simulink model "Fuzzy_intersection"  (R2025b)
settings: Solver=VariableStepAuto  StartTime=0.0  StopTime=100.0  RelTol=1e-3
model workspace (MAT data in the model file):
  RoadCapacity1 = 10
  RoadCapacity2 = 10
  RoadCapacity3 = 10
  RoadCapacity4 = 10
  TrafficControl : mamfis (value not decoded)
undefined symbols (not defined in the file or in its folder): m, n
libraries: fuzblock x2
settings Model: Creator=gyorgy  LastModifiedBy=gyorgy

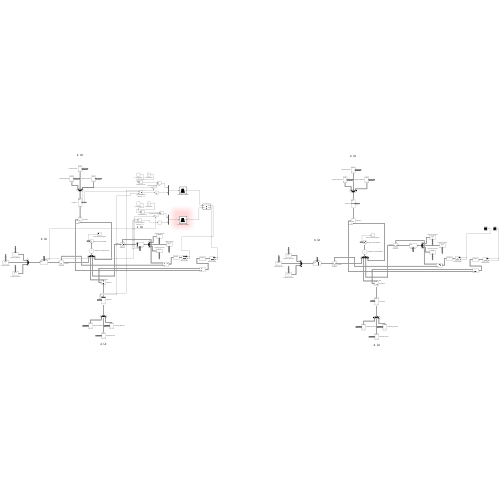
[thumbnail: Simulink's stored preview of the top-level diagram]
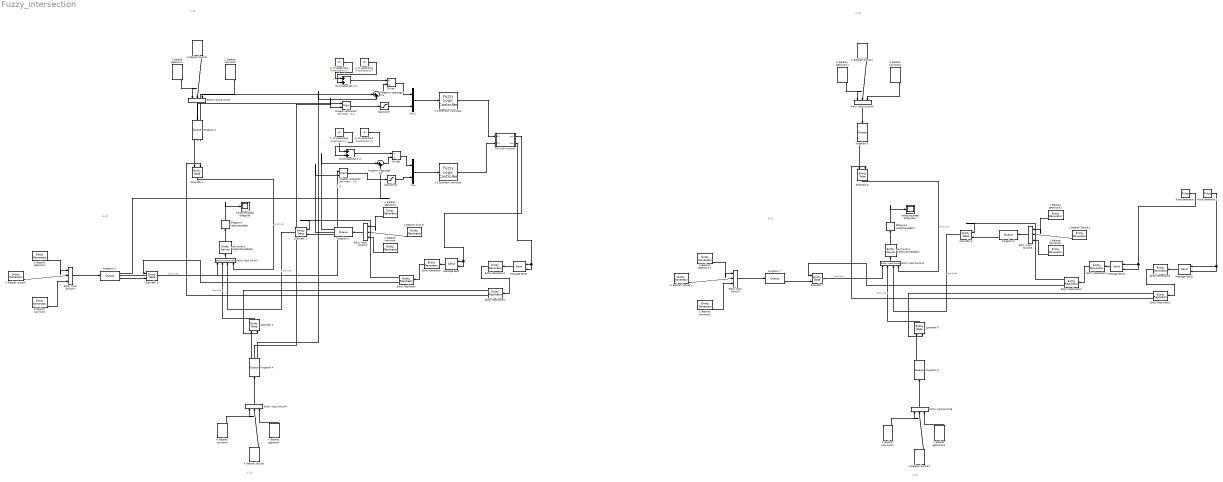
== system Fuzzy_intersection ==
  note: 1. Út
  note: 2. Út
  note: 3. Út
  note: 4. Út
  note: 3. Út
  note: 2. Út
  note: 4. Út
  1-3 Szemafor irányítása : fuzblock/Fuzzy Logic  Controller  FIS=TrafficControl  OutputSampleNumber=101  DataType=double  UseLookupTable=off  NumBreakpoints=10  FuzzifiedInputs=off  RuleFiringStrengths=off  RuleOutputs=off  AggregatedOutputs=off  SimulateUsing=Interpreted execution  OutOfRangeInputValueMessage=warning  NoRuleFiredMessage=warning  EmptyOutputFuzzySetMessage=warning
  1. Bejárat: buszok : EntityGenerator  OutputPortMessageModes=n,n,n,m  TimeSource=MATLAB action  IntergenerationTimeAction=|  GenerateEntityAtSimulationStart=off  GenerateAction=|  AttributeName=Utasok  NumberEntitiesDeparted=on  PendingEntityInBlock=on  AverageIntergenerationTime=on  EntityType=Structured  EntityTypeName=Jarmu
      | persistent rngInit;
      | if isempty(rngInit)
      |     seed = 11111;
      |     rng(seed);
      |     rngInit = true;
      | end
      | a = 1;
      | b = 20;
      | dt = a + (b-a).*rand(1,1);
      | persistent rngInit;
      | if isempty(rngInit)
      |     seed = 11111;
      |     rng(seed);
      |     rngInit = true;
      | end
      | 
      | % Pattern: Gaussian (normal) distribution
      | % m: Mean, d: Standard deviation
      | minpassengers = 1;
      | maxpassengers = 60;
      | m = 0; d = 0.2;
      | entity.Utasok = minpassengers + round((maxpassengers-minpassengers) * abs(m + d * randn));
      settings: OutputPortMap=o0,o1,o2,o3
  1. Bejárat: buszok1 : EntityGenerator  OutputPortMessageModes=n,n,n,m  TimeSource=MATLAB action  IntergenerationTimeAction=|  GenerateEntityAtSimulationStart=off  GenerateAction=|  AttributeName=Utasok  NumberEntitiesDeparted=on  PendingEntityInBlock=on  AverageIntergenerationTime=on  EntityType=Structured  EntityTypeName=Jarmu
      | persistent rngInit;
      | if isempty(rngInit)
      |     seed = 11111;
      |     rng(seed);
      |     rngInit = true;
      | end
      | a = 1;
      | b = 20;
      | dt = a + (b-a).*rand(1,1);
      | persistent rngInit;
      | if isempty(rngInit)
      |     seed = 11111;
      |     rng(seed);
      |     rngInit = true;
      | end
      | 
      | % Pattern: Gaussian (normal) distribution
      | % m: Mean, d: Standard deviation
      | minpassengers = 1;
      | maxpassengers = 60;
      | m = 0; d = 0.2;
      | entity.Utasok = minpassengers + round((maxpassengers-minpassengers) * abs(m + d * randn));
      settings: OutputPortMap=o0,o1,o2,o3
  1. Bejárat: gépkocsik : EntityGenerator  OutputPortMessageModes=n,n,n,m  TimeSource=MATLAB action  Period=0.1  IntergenerationTimeAction=|  GenerateEntityAtSimulationStart=off  GenerateAction=|  AttributeName=Utasok  NumberEntitiesDeparted=on  PendingEntityInBlock=on  AverageIntergenerationTime=on  EntityType=Structured  EntityTypeName=Jarmu
      | persistent rngInit;
      | if isempty(rngInit)
      |     seed = 11111;
      |     rng(seed);
      |     rngInit = true;
      | end
      | a = 1;
      | b = 5;
      | dt = a + (b-a).*rand(1,1);
      | persistent rngInit;
      | if isempty(rngInit)
      |     seed = 11111;
      |     rng(seed);
      |     rngInit = true;
      | end
      | 
      | % Pattern: Gaussian (normal) distribution
      | % m: Mean, d: Standard deviation
      | minpassengers = 1;
      | maxpassengers = 5;
      | m = 0; d = 0.2;
      | entity.Utasok = minpassengers + round((maxpassengers-minpassengers) * abs(m + d * randn));
      settings: OutputPortMap=o0,o1,o2,o3
  1. Bejárat: gépkocsik1 : EntityGenerator  OutputPortMessageModes=n,n,n,m  TimeSource=MATLAB action  Period=0.1  IntergenerationTimeAction=|  GenerateEntityAtSimulationStart=off  GenerateAction=|  AttributeName=Utasok  NumberEntitiesDeparted=on  PendingEntityInBlock=on  AverageIntergenerationTime=on  EntityType=Structured  EntityTypeName=Jarmu
      | persistent rngInit;
      | if isempty(rngInit)
      |     seed = 11111;
      |     rng(seed);
      |     rngInit = true;
      | end
      | a = 1;
      | b = 5;
      | dt = a + (b-a).*rand(1,1);
      | persistent rngInit;
      | if isempty(rngInit)
      |     seed = 11111;
      |     rng(seed);
      |     rngInit = true;
      | end
      | 
      | % Pattern: Gaussian (normal) distribution
      | % m: Mean, d: Standard deviation
      | minpassengers = 1;
      | maxpassengers = 5;
      | m = 0; d = 0.2;
      | entity.Utasok = minpassengers + round((maxpassengers-minpassengers) * abs(m + d * randn));
      settings: OutputPortMap=o0,o1,o2,o3
  1. Bejárat: kamionok : EntityGenerator  OutputPortMessageModes=n,n,n,m  TimeSource=MATLAB action  IntergenerationTimeAction=|  GenerateEntityAtSimulationStart=off  GenerateAction=|  AttributeName=Utasok  NumberEntitiesDeparted=on  PendingEntityInBlock=on  AverageIntergenerationTime=on  EntityType=Structured  EntityTypeName=Jarmu  DataInitialValue=1
      | persistent rngInit;
      | if isempty(rngInit)
      |     seed = 11111;
      |     rng(seed);
      |     rngInit = true;
      | end
      | a = 1;
      | b = 10;
      | dt = a + (b-a).*rand(1,1);
      | persistent rngInit;
      | if isempty(rngInit)
      |     seed = 11111;
      |     rng(seed);
      |     rngInit = true;
      | end
      | 
      | % Pattern: Gaussian (normal) distribution
      | % m: Mean, d: Standard deviation
      | minpassengers = 1;
      | maxpassengers = 2;
      | m = 0; d = 0.2;
      | entity.Utasok = minpassengers + round((maxpassengers-minpassengers) * abs(m + d * randn));
      settings: OutputPortMap=o0,o1,o2,o3
  1. Bejárat: kamionok1 : EntityGenerator  OutputPortMessageModes=n,n,n,m  TimeSource=MATLAB action  IntergenerationTimeAction=|  GenerateEntityAtSimulationStart=off  GenerateAction=|  AttributeName=Utasok  NumberEntitiesDeparted=on  PendingEntityInBlock=on  AverageIntergenerationTime=on  EntityType=Structured  EntityTypeName=Jarmu  DataInitialValue=1
      | persistent rngInit;
      | if isempty(rngInit)
      |     seed = 11111;
      |     rng(seed);
      |     rngInit = true;
      | end
      | a = 1;
      | b = 10;
      | dt = a + (b-a).*rand(1,1);
      | persistent rngInit;
      | if isempty(rngInit)
      |     seed = 11111;
      |     rng(seed);
      |     rngInit = true;
      | end
      | 
      | % Pattern: Gaussian (normal) distribution
      | % m: Mean, d: Standard deviation
      | minpassengers = 1;
      | maxpassengers = 2;
      | m = 0; d = 0.2;
      | entity.Utasok = minpassengers + round((maxpassengers-minpassengers) * abs(m + d * randn));
      settings: OutputPortMap=o0,o1,o2,o3
  "1. út kapacitása " : Constant  Value=RoadCapacity1
  2-4 Szemafor irányítása : fuzblock/Fuzzy Logic  Controller  FIS=TrafficControl  OutputSampleNumber=101  DataType=double  UseLookupTable=off  NumBreakpoints=10  FuzzifiedInputs=off  RuleFiringStrengths=off  RuleOutputs=off  AggregatedOutputs=off  SimulateUsing=Interpreted execution  OutOfRangeInputValueMessage=warning  NoRuleFiredMessage=warning  EmptyOutputFuzzySetMessage=warning
  2. Bejárat: buszok : EntityGenerator  OutputPortMessageModes=n,n,n,m  TimeSource=MATLAB action  IntergenerationTimeAction=|  GenerateEntityAtSimulationStart=off  GenerateAction=|  AttributeName=Utasok  NumberEntitiesDeparted=on  PendingEntityInBlock=on  AverageIntergenerationTime=on  EntityType=Structured  EntityTypeName=Jarmu
      | persistent rngInit;
      | if isempty(rngInit)
      |     seed = 22222;
      |     rng(seed);
      |     rngInit = true;
      | end
      | a = 1;
      | b = 20;
      | dt = a + (b-a).*rand(1,1);
      | persistent rngInit;
      | if isempty(rngInit)
      |     seed = 22222;
      |     rng(seed);
      |     rngInit = true;
      | end
      | 
      | % Pattern: Gaussian (normal) distribution
      | % m: Mean, d: Standard deviation
      | minpassengers = 1;
      | maxpassengers = 60;
      | m = 0; d = 0.2;
      | entity.Utasok = minpassengers + round((maxpassengers-minpassengers) * abs(m + d * randn));
      settings: OutputPortMap=o0,o1,o2,o3
  2. Bejárat: buszok1 : EntityGenerator  OutputPortMessageModes=n,n,n,m  TimeSource=MATLAB action  IntergenerationTimeAction=|  GenerateEntityAtSimulationStart=off  GenerateAction=|  AttributeName=Utasok  NumberEntitiesDeparted=on  PendingEntityInBlock=on  AverageIntergenerationTime=on  EntityType=Structured  EntityTypeName=Jarmu
      | persistent rngInit;
      | if isempty(rngInit)
      |     seed = 22222;
      |     rng(seed);
      |     rngInit = true;
      | end
      | a = 1;
      | b = 20;
      | dt = a + (b-a).*rand(1,1);
      | persistent rngInit;
      | if isempty(rngInit)
      |     seed = 22222;
      |     rng(seed);
      |     rngInit = true;
      | end
      | 
      | % Pattern: Gaussian (normal) distribution
      | % m: Mean, d: Standard deviation
      | minpassengers = 1;
      | maxpassengers = 60;
      | m = 0; d = 0.2;
      | entity.Utasok = minpassengers + round((maxpassengers-minpassengers) * abs(m + d * randn));
      settings: OutputPortMap=o0,o1,o2,o3
  2. Bejárat: gépkocsik : EntityGenerator  OutputPortMessageModes=n,n,n,m  TimeSource=MATLAB action  Period=0.1  IntergenerationTimeAction=|  GenerateEntityAtSimulationStart=off  GenerateAction=|  AttributeName=Utasok  NumberEntitiesDeparted=on  PendingEntityInBlock=on  AverageIntergenerationTime=on  EntityType=Structured  EntityTypeName=Jarmu
      | persistent rngInit;
      | if isempty(rngInit)
      |     seed = 22222;
      |     rng(seed);
      |     rngInit = true;
      | end
      | a = 1;
      | b = 5;
      | dt = a + (b-a).*rand(1,1);
      | persistent rngInit;
      | if isempty(rngInit)
      |     seed = 22222;
      |     rng(seed);
      |     rngInit = true;
      | end
      | 
      | % Pattern: Gaussian (normal) distribution
      | % m: Mean, d: Standard deviation
      | minpassengers = 1;
      | maxpassengers = 5;
      | m = 0; d = 0.2;
      | entity.Utasok = minpassengers + round((maxpassengers-minpassengers) * abs(m + d * randn));
      settings: OutputPortMap=o0,o1,o2,o3
  2. Bejárat: gépkocsik1 : EntityGenerator  OutputPortMessageModes=n,n,n,m  TimeSource=MATLAB action  Period=0.1  IntergenerationTimeAction=|  GenerateEntityAtSimulationStart=off  GenerateAction=|  AttributeName=Utasok  NumberEntitiesDeparted=on  PendingEntityInBlock=on  AverageIntergenerationTime=on  EntityType=Structured  EntityTypeName=Jarmu
      | persistent rngInit;
      | if isempty(rngInit)
      |     seed = 22222;
      |     rng(seed);
      |     rngInit = true;
      | end
      | a = 1;
      | b = 5;
      | dt = a + (b-a).*rand(1,1);
      | persistent rngInit;
      | if isempty(rngInit)
      |     seed = 22222;
      |     rng(seed);
      |     rngInit = true;
      | end
      | 
      | % Pattern: Gaussian (normal) distribution
      | % m: Mean, d: Standard deviation
      | minpassengers = 1;
      | maxpassengers = 5;
      | m = 0; d = 0.2;
      | entity.Utasok = minpassengers + round((maxpassengers-minpassengers) * abs(m + d * randn));
      settings: OutputPortMap=o0,o1,o2,o3
  2. Bejárat: kamionok : EntityGenerator  OutputPortMessageModes=n,n,n,m  TimeSource=MATLAB action  IntergenerationTimeAction=|  GenerateEntityAtSimulationStart=off  GenerateAction=|  AttributeName=Utasok  NumberEntitiesDeparted=on  PendingEntityInBlock=on  AverageIntergenerationTime=on  EntityType=Structured  EntityTypeName=Jarmu
      | persistent rngInit;
      | if isempty(rngInit)
      |     seed = 22222;
      |     rng(seed);
      |     rngInit = true;
      | end
      | a = 1;
      | b = 10;
      | dt = a + (b-a).*rand(1,1);
      | persistent rngInit;
      | if isempty(rngInit)
      |     seed = 22222;
      |     rng(seed);
      |     rngInit = true;
      | end
      | 
      | % Pattern: Gaussian (normal) distribution
      | % m: Mean, d: Standard deviation
      | minpassengers = 1;
      | maxpassengers = 2;
      | m = 0; d = 0.2;
      | entity.Utasok = minpassengers + round((maxpassengers-minpassengers) * abs(m + d * randn));
      settings: OutputPortMap=o0,o1,o2,o3
  2. Bejárat: kamionok1 : EntityGenerator  OutputPortMessageModes=n,n,n,m  TimeSource=MATLAB action  IntergenerationTimeAction=|  GenerateEntityAtSimulationStart=off  GenerateAction=|  AttributeName=Utasok  NumberEntitiesDeparted=on  PendingEntityInBlock=on  AverageIntergenerationTime=on  EntityType=Structured  EntityTypeName=Jarmu
      | persistent rngInit;
      | if isempty(rngInit)
      |     seed = 22222;
      |     rng(seed);
      |     rngInit = true;
      | end
      | a = 1;
      | b = 10;
      | dt = a + (b-a).*rand(1,1);
      | persistent rngInit;
      | if isempty(rngInit)
      |     seed = 22222;
      |     rng(seed);
      |     rngInit = true;
      | end
      | 
      | % Pattern: Gaussian (normal) distribution
      | % m: Mean, d: Standard deviation
      | minpassengers = 1;
      | maxpassengers = 2;
      | m = 0; d = 0.2;
      | entity.Utasok = minpassengers + round((maxpassengers-minpassengers) * abs(m + d * randn));
      settings: OutputPortMap=o0,o1,o2,o3
  2. út kapacitása : Constant  Value=RoadCapacity2
  3. Bejárat: buszok : EntityGenerator  OutputPortMessageModes=n,n,n,m  TimeSource=MATLAB action  IntergenerationTimeAction=|  GenerateEntityAtSimulationStart=off  GenerateAction=|  AttributeName=Utasok  NumberEntitiesDeparted=on  PendingEntityInBlock=on  AverageIntergenerationTime=on  EntityType=Structured  EntityTypeName=Jarmu
      | persistent rngInit;
      | if isempty(rngInit)
      |     seed = 33333;
      |     rng(seed);
      |     rngInit = true;
      | end
      | a = 1;
      | b = 20;
      | dt = a + (b-a).*rand(1,1);
      | persistent rngInit;
      | if isempty(rngInit)
      |     seed = 33333;
      |     rng(seed);
      |     rngInit = true;
      | end
      | 
      | % Pattern: Gaussian (normal) distribution
      | % m: Mean, d: Standard deviation
      | minpassengers = 1;
      | maxpassengers = 60;
      | m = 0; d = 0.2;
      | entity.Utasok = minpassengers + round((maxpassengers-minpassengers) * abs(m + d * randn));
      settings: OutputPortMap=o0,o1,o2,o3
  3. Bejárat: buszok1 : EntityGenerator  OutputPortMessageModes=n,n,n,m  TimeSource=MATLAB action  IntergenerationTimeAction=|  GenerateEntityAtSimulationStart=off  GenerateAction=|  AttributeName=Utasok  NumberEntitiesDeparted=on  PendingEntityInBlock=on  AverageIntergenerationTime=on  EntityType=Structured  EntityTypeName=Jarmu
      | persistent rngInit;
      | if isempty(rngInit)
      |     seed = 33333;
      |     rng(seed);
      |     rngInit = true;
      | end
      | a = 1;
      | b = 20;
      | dt = a + (b-a).*rand(1,1);
      | persistent rngInit;
      | if isempty(rngInit)
      |     seed = 33333;
      |     rng(seed);
      |     rngInit = true;
      | end
      | 
      | % Pattern: Gaussian (normal) distribution
      | % m: Mean, d: Standard deviation
      | minpassengers = 1;
      | maxpassengers = 60;
      | m = 0; d = 0.2;
      | entity.Utasok = minpassengers + round((maxpassengers-minpassengers) * abs(m + d * randn));
      settings: OutputPortMap=o0,o1,o2,o3
  3. Bejárat: gépkocsik : EntityGenerator  OutputPortMessageModes=n,n,n,m  TimeSource=MATLAB action  Period=0.1  IntergenerationTimeAction=|  GenerateEntityAtSimulationStart=off  GenerateAction=|  AttributeName=Utasok  NumberEntitiesDeparted=on  PendingEntityInBlock=on  AverageIntergenerationTime=on  EntityType=Structured  EntityTypeName=Jarmu
      | persistent rngInit;
      | if isempty(rngInit)
      |     seed = 33333;
      |     rng(seed);
      |     rngInit = true;
      | end
      | a = 1;
      | b = 5;
      | dt = a + (b-a).*rand(1,1);
      | persistent rngInit;
      | if isempty(rngInit)
      |     seed = 33333;
      |     rng(seed);
      |     rngInit = true;
      | end
      | 
      | % Pattern: Gaussian (normal) distribution
      | % m: Mean, d: Standard deviation
      | minpassengers = 1;
      | maxpassengers = 5;
      | m = 0; d = 0.2;
      | entity.Utasok = minpassengers + round((maxpassengers-minpassengers) * abs(m + d * randn));
      settings: OutputPortMap=o0,o1,o2,o3
  3. Bejárat: gépkocsik1 : EntityGenerator  OutputPortMessageModes=n,n,n,m  TimeSource=MATLAB action  Period=0.1  IntergenerationTimeAction=|  GenerateEntityAtSimulationStart=off  GenerateAction=|  AttributeName=Utasok  NumberEntitiesDeparted=on  PendingEntityInBlock=on  AverageIntergenerationTime=on  EntityType=Structured  EntityTypeName=Jarmu
      | persistent rngInit;
      | if isempty(rngInit)
      |     seed = 33333;
      |     rng(seed);
      |     rngInit = true;
      | end
      | a = 1;
      | b = 5;
      | dt = a + (b-a).*rand(1,1);
      | persistent rngInit;
      | if isempty(rngInit)
      |     seed = 33333;
      |     rng(seed);
      |     rngInit = true;
      | end
      | 
      | % Pattern: Gaussian (normal) distribution
      | % m: Mean, d: Standard deviation
      | minpassengers = 1;
      | maxpassengers = 5;
      | m = 0; d = 0.2;
      | entity.Utasok = minpassengers + round((maxpassengers-minpassengers) * abs(m + d * randn));
      settings: OutputPortMap=o0,o1,o2,o3
  3. Bejárat: kamionok : EntityGenerator  OutputPortMessageModes=n,n,n,m  TimeSource=MATLAB action  IntergenerationTimeAction=|  GenerateEntityAtSimulationStart=off  GenerateAction=|  AttributeName=Utasok  NumberEntitiesDeparted=on  PendingEntityInBlock=on  AverageIntergenerationTime=on  EntityType=Structured  EntityTypeName=Jarmu
      | persistent rngInit;
      | if isempty(rngInit)
      |     seed = 33333;
      |     rng(seed);
      |     rngInit = true;
      | end
      | a = 1;
      | b = 10;
      | dt = a + (b-a).*rand(1,1);
      | persistent rngInit;
      | if isempty(rngInit)
      |     seed = 33333;
      |     rng(seed);
      |     rngInit = true;
      | end
      | 
      | % Pattern: Gaussian (normal) distribution
      | % m: Mean, d: Standard deviation
      | minpassengers = 1;
      | maxpassengers = 2;
      | m = 0; d = 0.2;
      | entity.Utasok = minpassengers + round((maxpassengers-minpassengers) * abs(m + d * randn));
      settings: OutputPortMap=o0,o1,o2,o3
  3. Bejárat: kamionok1 : EntityGenerator  OutputPortMessageModes=n,n,n,m  TimeSource=MATLAB action  IntergenerationTimeAction=|  GenerateEntityAtSimulationStart=off  GenerateAction=|  AttributeName=Utasok  NumberEntitiesDeparted=on  PendingEntityInBlock=on  AverageIntergenerationTime=on  EntityType=Structured  EntityTypeName=Jarmu
      | persistent rngInit;
      | if isempty(rngInit)
      |     seed = 33333;
      |     rng(seed);
      |     rngInit = true;
      | end
      | a = 1;
      | b = 10;
      | dt = a + (b-a).*rand(1,1);
      | persistent rngInit;
      | if isempty(rngInit)
      |     seed = 33333;
      |     rng(seed);
      |     rngInit = true;
      | end
      | 
      | % Pattern: Gaussian (normal) distribution
      | % m: Mean, d: Standard deviation
      | minpassengers = 1;
      | maxpassengers = 2;
      | m = 0; d = 0.2;
      | entity.Utasok = minpassengers + round((maxpassengers-minpassengers) * abs(m + d * randn));
      settings: OutputPortMap=o0,o1,o2,o3
  3. út kapacitása : Constant  Value=RoadCapacity3
  4. Bejárat: buszok : EntityGenerator  OutputPortMessageModes=n,n,n,m  TimeSource=MATLAB action  IntergenerationTimeAction=|  GenerateEntityAtSimulationStart=off  GenerateAction=|  AttributeName=Utasok  NumberEntitiesDeparted=on  PendingEntityInBlock=on  AverageIntergenerationTime=on  EntityType=Structured  EntityTypeName=Jarmu
      | persistent rngInit;
      | if isempty(rngInit)
      |     seed = 44444;
      |     rng(seed);
      |     rngInit = true;
      | end
      | a = 1;
      | b = 20;
      | dt = a + (b-a).*rand(1,1);
      | persistent rngInit;
      | if isempty(rngInit)
      |     seed = 44444;
      |     rng(seed);
      |     rngInit = true;
      | end
      | 
      | % Pattern: Gaussian (normal) distribution
      | % m: Mean, d: Standard deviation
      | minpassengers = 1;
      | maxpassengers = 60;
      | m = 0; d = 0.2;
      | entity.Utasok = minpassengers + round((maxpassengers-minpassengers) * abs(m + d * randn));
      settings: OutputPortMap=o0,o1,o2,o3
  4. Bejárat: buszok1 : EntityGenerator  OutputPortMessageModes=n,n,n,m  TimeSource=MATLAB action  IntergenerationTimeAction=|  GenerateEntityAtSimulationStart=off  GenerateAction=|  AttributeName=Utasok  NumberEntitiesDeparted=on  PendingEntityInBlock=on  AverageIntergenerationTime=on  EntityType=Structured  EntityTypeName=Jarmu
      | persistent rngInit;
      | if isempty(rngInit)
      |     seed = 44444;
      |     rng(seed);
      |     rngInit = true;
      | end
      | a = 1;
      | b = 20;
      | dt = a + (b-a).*rand(1,1);
      | persistent rngInit;
      | if isempty(rngInit)
      |     seed = 44444;
      |     rng(seed);
      |     rngInit = true;
      | end
      | 
      | % Pattern: Gaussian (normal) distribution
      | % m: Mean, d: Standard deviation
      | minpassengers = 1;
      | maxpassengers = 60;
      | m = 0; d = 0.2;
      | entity.Utasok = minpassengers + round((maxpassengers-minpassengers) * abs(m + d * randn));
      settings: OutputPortMap=o0,o1,o2,o3
  4. Bejárat: gépkocsik : EntityGenerator  OutputPortMessageModes=n,n,n,m  TimeSource=MATLAB action  Period=0.1  IntergenerationTimeAction=|  GenerateEntityAtSimulationStart=off  GenerateAction=|  AttributeName=Utasok  NumberEntitiesDeparted=on  PendingEntityInBlock=on  AverageIntergenerationTime=on  EntityType=Structured  EntityTypeName=Jarmu
      | persistent rngInit;
      | if isempty(rngInit)
      |     seed = 44444;
      |     rng(seed);
      |     rngInit = true;
      | end
      | a = 1;
      | b = 5;
      | dt = a + (b-a).*rand(1,1);
      | persistent rngInit;
      | if isempty(rngInit)
      |     seed = 44444;
      |     rng(seed);
      |     rngInit = true;
      | end
      | 
      | % Pattern: Gaussian (normal) distribution
      | % m: Mean, d: Standard deviation
      | minpassengers = 1;
      | maxpassengers = 5;
      | m = 0; d = 0.2;
      | entity.Utasok = minpassengers + round((maxpassengers-minpassengers) * abs(m + d * randn));
      settings: OutputPortMap=o0,o1,o2,o3
  4. Bejárat: gépkocsik1 : EntityGenerator  OutputPortMessageModes=n,n,n,m  TimeSource=MATLAB action  Period=0.1  IntergenerationTimeAction=|  GenerateEntityAtSimulationStart=off  GenerateAction=|  AttributeName=Utasok  NumberEntitiesDeparted=on  PendingEntityInBlock=on  AverageIntergenerationTime=on  EntityType=Structured  EntityTypeName=Jarmu
      | persistent rngInit;
      | if isempty(rngInit)
      |     seed = 44444;
      |     rng(seed);
      |     rngInit = true;
      | end
      | a = 1;
      | b = 5;
      | dt = a + (b-a).*rand(1,1);
      | persistent rngInit;
      | if isempty(rngInit)
      |     seed = 44444;
      |     rng(seed);
      |     rngInit = true;
      | end
      | 
      | % Pattern: Gaussian (normal) distribution
      | % m: Mean, d: Standard deviation
      | minpassengers = 1;
      | maxpassengers = 5;
      | m = 0; d = 0.2;
      | entity.Utasok = minpassengers + round((maxpassengers-minpassengers) * abs(m + d * randn));
      settings: OutputPortMap=o0,o1,o2,o3
  4. Bejárat: kamionok : EntityGenerator  OutputPortMessageModes=n,n,n,m  TimeSource=MATLAB action  IntergenerationTimeAction=|  GenerateEntityAtSimulationStart=off  GenerateAction=|  AttributeName=Utasok  NumberEntitiesDeparted=on  PendingEntityInBlock=on  AverageIntergenerationTime=on  EntityType=Structured  EntityTypeName=Jarmu
      | persistent rngInit;
      | if isempty(rngInit)
      |     seed = 44444;
      |     rng(seed);
      |     rngInit = true;
      | end
      | a = 1;
      | b = 10;
      | dt = a + (b-a).*rand(1,1);
      | persistent rngInit;
      | if isempty(rngInit)
      |     seed = 44444;
      |     rng(seed);
      |     rngInit = true;
      | end
      | 
      | % Pattern: Gaussian (normal) distribution
      | % m: Mean, d: Standard deviation
      | minpassengers = 1;
      | maxpassengers = 2;
      | m = 0; d = 0.2;
      | entity.Utasok = minpassengers + round((maxpassengers-minpassengers) * abs(m + d * randn));
      settings: OutputPortMap=o0,o1,o2,o3
  4. Bejárat: kamionok1 : EntityGenerator  OutputPortMessageModes=n,n,n,m  TimeSource=MATLAB action  IntergenerationTimeAction=|  GenerateEntityAtSimulationStart=off  GenerateAction=|  AttributeName=Utasok  NumberEntitiesDeparted=on  PendingEntityInBlock=on  AverageIntergenerationTime=on  EntityType=Structured  EntityTypeName=Jarmu
      | persistent rngInit;
      | if isempty(rngInit)
      |     seed = 44444;
      |     rng(seed);
      |     rngInit = true;
      | end
      | a = 1;
      | b = 10;
      | dt = a + (b-a).*rand(1,1);
      | persistent rngInit;
      | if isempty(rngInit)
      |     seed = 44444;
      |     rng(seed);
      |     rngInit = true;
      | end
      | 
      | % Pattern: Gaussian (normal) distribution
      | % m: Mean, d: Standard deviation
      | minpassengers = 1;
      | maxpassengers = 2;
      | m = 0; d = 0.2;
      | entity.Utasok = minpassengers + round((maxpassengers-minpassengers) * abs(m + d * randn));
      settings: OutputPortMap=o0,o1,o2,o3
  4. út kapacitása : Constant  Value=RoadCapacity4
  Atlagos várakozási idő (max) - 1-3 : MinMax  Function=max  Inputs=2
  Atlagos várakozási idő (max) - 2-4 : MinMax  Function=max  Inputs=2  OutDataTypeStr=double
  Divide : Product  Inputs=/*
  Divide1 : Product  Inputs=/*  InputSameDT=on  OutDataTypeStr=double
  Elhagyja a kereszteződést : EntityTerminator  InputPortMessageModes=m  NumberEntitiesArrived=on
      settings: OutputPortMap=o0
  Elhagyja a kereszteződést1 : EntityTerminator  InputPortMessageModes=m  NumberEntitiesArrived=on
      settings: OutputPortMap=o0
  Entity Input Switch : EntityInputSwitch  InputPortMessageModes=m,m,m,m  OutputPortMessageModes=m  NumberInputPorts=4
      settings: InputPortMap=u1,u2,u3,u4
  Entity Input Switch1 : EntityInputSwitch  InputPortMessageModes=m,m,m,m  OutputPortMessageModes=m  NumberInputPorts=4
      settings: InputPortMap=u1,u2,u3,u4
  Entity Input Switch{2..9} (8 alike) : EntityInputSwitch  InputPortMessageModes=m,m,m  OutputPortMessageModes=m  NumberInputPorts=3
      settings: InputPortMap=u1,u2,u3
  Entity Generator{,1..3} (4 alike) : EntityGenerator  InputPortMessageModes=m  OutputPortMessageModes=m  GenerationMethod=Event-based  TimeSource=Signal port  AttributeName=entity  EntityTypeName=Entity  DataInitialValue=1
      settings: InputPortMap=u0
  Entity Replicator : EntityReplicator  InputPortMessageModes=m  OutputPortMessageModes=m,m  ReplicasDepartFrom=Single output port  NumberReplicas=2  HoldOriginalEntityUntilAllReplicasDepart=on
  Entity Replicator1 : EntityReplicator  InputPortMessageModes=m  OutputPortMessageModes=m,m  ReplicasDepartFrom=Single output port  NumberReplicas=2
  Entity Replicator2 : EntityReplicator  InputPortMessageModes=m  OutputPortMessageModes=m,m  ReplicasDepartFrom=Single output port  NumberReplicas=2  HoldOriginalEntityUntilAllReplicasDepart=on
  Entity Replicator3 : EntityReplicator  InputPortMessageModes=m  OutputPortMessageModes=m,m  ReplicasDepartFrom=Single output port  NumberReplicas=2
  Forgalom 1 : Queue  InputPortMessageModes=m  OutputPortMessageModes=n,n,m  Capacity=RoadCapacity1  NumberEntitiesInBlock=on  AverageWait=on
      settings: OutputPortMap=o1,o2,o5
  Forgalom 2 : Queue  InputPortMessageModes=m  OutputPortMessageModes=n,n,m  Capacity=RoadCapacity2  NumberEntitiesInBlock=on  AverageWait=on
      settings: OutputPortMap=o1,o2,o5
  Forgalom 3 : Queue  InputPortMessageModes=m  OutputPortMessageModes=n,n,m  Capacity=RoadCapacity3  NumberEntitiesInBlock=on  AverageWait=on
      settings: OutputPortMap=o1,o2,o5
  Forgalom 4 : Queue  InputPortMessageModes=m  OutputPortMessageModes=n,n,m  Capacity=RoadCapacity4  NumberEntitiesInBlock=on  AverageWait=on
      settings: OutputPortMap=o1,o2,o5
  Forgalom 5 : Queue  InputPortMessageModes=m  OutputPortMessageModes=n,n,m  Capacity=RoadCapacity1  NumberEntitiesInBlock=on  AverageWait=on
      settings: OutputPortMap=o1,o2,o5
  Forgalom 6 : Queue  InputPortMessageModes=m  OutputPortMessageModes=n,n,m  Capacity=RoadCapacity2  NumberEntitiesInBlock=on  AverageWait=on
      settings: OutputPortMap=o1,o2,o5
  Forgalom 7 : Queue  InputPortMessageModes=m  OutputPortMessageModes=n,n,m  Capacity=RoadCapacity3  NumberEntitiesInBlock=on  AverageWait=on
      settings: OutputPortMap=o1,o2,o5
  Forgalom 8 : Queue  InputPortMessageModes=m  OutputPortMessageModes=n,n,m  Capacity=RoadCapacity4  NumberEntitiesInBlock=on  AverageWait=on
      settings: OutputPortMap=o1,o2,o5
  Forgalom nagysága - 1-3 : Sum  Inputs=|++
  Forgalom nagysága - 2-4 : Sum  Inputs=|++
  Járművek a keresztezodésben : EntityServer  InputPortMessageModes=m  OutputPortMessageModes=m  Capacity=2  ServiceTimeSource=MATLAB action  ServiceTimeAction=|
      | persistent rngInit;
      | if isempty(rngInit)
      |     seed = 55555;
      |     rng(seed);
      |     rngInit = true;
      | end
      | 
      | % Pattern: Gaussian (normal) distribution
      | % m: Mean, d: Standard deviation
      | m = 0; d = 1;
      | dt = abs(m + d * randn);
  Járművek a keresztezodésben1 : EntityServer  InputPortMessageModes=m  OutputPortMessageModes=m  Capacity=2  ServiceTimeSource=MATLAB action  ServiceTimeAction=|
      | persistent rngInit;
      | if isempty(rngInit)
      |     seed = 55555;
      |     rng(seed);
      |     rngInit = true;
      | end
      | 
      | % Pattern: Gaussian (normal) distribution
      | % m: Mean, d: Standard deviation
      | m = 0; d = 1;
      | dt = abs(m + d * randn);
  Kereszteződést elhagyták : Scope
      settings: ActiveDisplayYMinimum=227.06108147411885  ActiveDisplayYMaximum=238.86097723623857
  Kereszteződést elhagyták1 : Scope
      settings: ActiveDisplayYMinimum=222.88265852629056  ActiveDisplayYMaximum=223.04054883446648
  MATLAB Function : MATLAB Function  TreatAsAtomicUnit=on
  Message Send{,1..3} (4 alike) : Send  OutputPortMessageModes=m  ShowEnablePort=on
      settings: InputPortMap=e0,u1
  Mux : Mux  Inputs=2
  Mux1 : Mux  Inputs=2
  Pulse Generator : DiscretePulseGenerator  PulseType=Time based  Period=20  PulseWidth=50
  Pulse Generator1 : DiscretePulseGenerator  PulseType=Time based  Period=20  PulseWidth=50  PhaseDelay=10
  Saturation : Saturate  UpperLimit=30  LowerLimit=0  OutDataTypeStr=double
  Saturation1 : Saturate  UpperLimit=30  LowerLimit=0  OutDataTypeStr=double
  Szemafor {1..8} (8 alike) : EntityGate  InputPortMessageModes=m,m  OutputPortMessageModes=m
  Összkapacitás 1-3 : Sum
  Összkapacitás 2-4 : Sum
  wires:
  Forgalom 1/3 -> Szemafor 1/2
  Forgalom 2/3 -> Szemafor 2/2
  Forgalom 3/3 -> Szemafor 3/2
  Entity Input Switch3/1 -> Forgalom 3/1
  Forgalom 4/3 -> Szemafor 4/2
  Entity Input Switch4/1 -> Forgalom 4/1
  Járművek a keresztezodésben/1 -> Elhagyja a kereszteződést/1
  Entity Input Switch/1 -> Járművek a keresztezodésben/1
  Szemafor 3/1 -> Entity Input Switch/1  "Járművek"
  Szemafor 4/1 -> Entity Input Switch/2  "Járművek"
  Szemafor 1/1 -> Entity Input Switch/3  "Járművek"
  Szemafor 2/1 -> Entity Input Switch/4  "Járművek"
  Entity Input Switch5/1 -> Forgalom 2/1
  1. Bejárat: gépkocsik/4 -> Entity Input Switch2/1
  1. Bejárat: buszok/4 -> Entity Input Switch2/2
  1. Bejárat: kamionok/4 -> Entity Input Switch2/3
  2. Bejárat: kamionok/4 -> Entity Input Switch5/3
  2. Bejárat: gépkocsik/4 -> Entity Input Switch5/1
  2. Bejárat: buszok/4 -> Entity Input Switch5/2
  3. Bejárat: buszok/4 -> Entity Input Switch3/2
  3. Bejárat: gépkocsik/4 -> Entity Input Switch3/1
  3. Bejárat: kamionok/4 -> Entity Input Switch3/3
  4. Bejárat: buszok/4 -> Entity Input Switch4/2
  4. Bejárat: gépkocsik/4 -> Entity Input Switch4/3
  4. Bejárat: kamionok/4 -> Entity Input Switch4/1
  Mux/1 -> 1-3 Szemafor irányítása/1
  Forgalom 1/2 -> Atlagos várakozási idő (max) - 1-3/2
  Forgalom 3/2 -> Atlagos várakozási idő (max) - 1-3/1
  Mux1/1 -> 2-4 Szemafor irányítása/1
  Forgalom 1/1 -> Forgalom nagysága - 1-3/1
  Forgalom 3/1 -> Forgalom nagysága - 1-3/2
  Forgalom 4/1 -> Forgalom nagysága - 2-4/2
  Forgalom 2/1 -> Forgalom nagysága - 2-4/1
  Entity Replicator/1 -> Szemafor 1/1
  Entity Replicator/2 -> Szemafor 3/1
  Entity Replicator1/1 -> Szemafor 4/1
  Entity Replicator1/2 -> Szemafor 2/1
  Entity Input Switch2/1 -> Forgalom 1/1
  Saturation/1 -> Mux1/2
  Saturation1/1 -> Mux/2
  Atlagos várakozási idő (max) - 1-3/1 -> Saturation1/1
  2. út kapacitása/1 -> Összkapacitás 2-4/1
  4. út kapacitása/1 -> Összkapacitás 2-4/2
  "1. út kapacitása "/1 -> Összkapacitás 1-3/1
  3. út kapacitása/1 -> Összkapacitás 1-3/2
  Forgalom nagysága - 2-4/1 -> Divide/2
  Összkapacitás 1-3/1 -> Divide1/1
  Divide1/1 -> Mux/1
  Összkapacitás 2-4/1 -> Divide/1
  Divide/1 -> Mux1/1
  Atlagos várakozási idő (max) - 2-4/1 -> Saturation/1
  Forgalom nagysága - 1-3/1 -> Divide1/2
  Forgalom 4/2 -> Atlagos várakozási idő (max) - 2-4/2
  Forgalom 2/2 -> Atlagos várakozási idő (max) - 2-4/1
  Entity Generator/1 -> Entity Replicator/1
  Entity Generator1/1 -> Entity Replicator1/1
  Message Send/1 -> Entity Generator/1
  MATLAB Function/1(sig1) -> Message Send/1, Message Send/2
  Message Send1/1 -> Entity Generator1/1
  MATLAB Function/2(sig2) -> Message Send1/1, Message Send1/2
  Elhagyja a kereszteződést/1 -> Kereszteződést elhagyták/1
  4. Bejárat: buszok1/4 -> Entity Input Switch8/2
  Járművek a keresztezodésben1/1 -> Elhagyja a kereszteződést1/1
  2. Bejárat: kamionok1/4 -> Entity Input Switch9/3
  2. Bejárat: gépkocsik1/4 -> Entity Input Switch9/1
  3. Bejárat: kamionok1/4 -> Entity Input Switch7/3
  Forgalom 5/3 -> Szemafor 5/2
  Entity Replicator3/1 -> Szemafor 8/1
  Entity Input Switch8/1 -> Forgalom 8/1
  Entity Replicator2/2 -> Szemafor 7/1
  1. Bejárat: kamionok1/4 -> Entity Input Switch6/3
  1. Bejárat: buszok1/4 -> Entity Input Switch6/2
  2. Bejárat: buszok1/4 -> Entity Input Switch9/2
  Entity Input Switch9/1 -> Forgalom 6/1
  Entity Input Switch1/1 -> Járművek a keresztezodésben1/1
  1. Bejárat: gépkocsik1/4 -> Entity Input Switch6/1
  4. Bejárat: gépkocsik1/4 -> Entity Input Switch8/3
  Szemafor 7/1 -> Entity Input Switch1/1  "Járművek"
  Entity Replicator2/1 -> Szemafor 5/1
  Message Send3/1 -> Entity Generator3/1
  3. Bejárat: gépkocsik1/4 -> Entity Input Switch7/1
  Forgalom 6/3 -> Szemafor 6/2
  Entity Input Switch6/1 -> Forgalom 5/1
  Szemafor 5/1 -> Entity Input Switch1/3  "Járművek"
  4. Bejárat: kamionok1/4 -> Entity Input Switch8/1
  Forgalom 8/3 -> Szemafor 8/2
  Message Send2/1 -> Entity Generator2/1
  Elhagyja a kereszteződést1/1 -> Kereszteződést elhagyták1/1
  Entity Input Switch7/1 -> Forgalom 7/1
  3. Bejárat: buszok1/4 -> Entity Input Switch7/2
  Entity Replicator3/2 -> Szemafor 6/1
  Forgalom 7/3 -> Szemafor 7/2
  Szemafor 8/1 -> Entity Input Switch1/2  "Járművek"
  Szemafor 6/1 -> Entity Input Switch1/4  "Járművek"
  Pulse Generator/1 -> Message Send2/2, Message Send2/1
  Pulse Generator1/1 -> Message Send3/2, Message Send3/1
  Entity Generator2/1 -> Entity Replicator2/1
  Entity Generator3/1 -> Entity Replicator3/1
  1-3 Szemafor irányítása/1 -> MATLAB Function/2(fo2)
  2-4 Szemafor irányítása/1 -> MATLAB Function/1(fo1)

== matlab function Fuzzy_intersection/MATLAB Function ==
  data: fo1 input; sig1 output; fo2 input; sig2 output
function [sig1,sig2] = fcn(fo1,fo2)

if fo1 < fo2
    sig1 = 1;
    sig2 = 0;
else
    sig1 = 0;
    sig2 = 1;
end
